simulink model "Controls"  (R2020b)
settings: Solver=VariableStepAuto  StartTime=0.0  StopTime=30  RelTol=1e-3
model workspace (MAT data in the model file):
  l1 = Simulink.Parameter
  l1.Value = 0.2
  l1.Description = '"Bicep length"'
  l1.DataType = 'auto'
  l1.Dimensions = [1 1]
  l2 = Simulink.Parameter
  l2.Value = 0.15
  l2.Description = '"Forearm length"'
  l2.DataType = 'auto'
  l2.Dimensions = [1 1]
settings Model: PacingRate=0.500000  OrderedModelArguments=off  Creator=Luke Bidulka  LastModifiedBy=ndroz

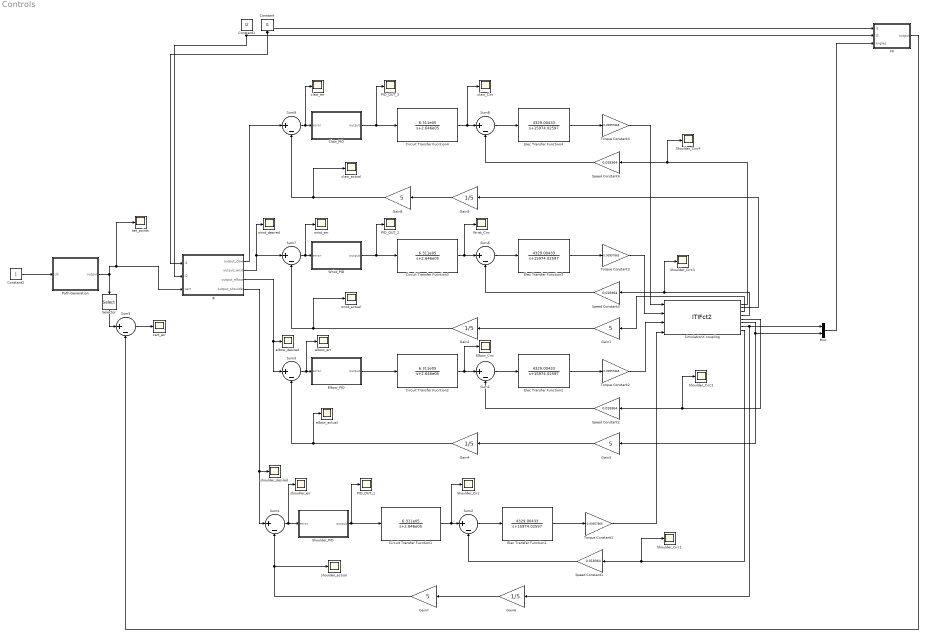
== system Controls ==
  Circuit Transfer Fucntion{1..4} (4 alike) : TransferFcn  Numerator=[6.311e05]  Denominator=[1 2.646e05]
  Claw_PID : MATLAB Function  TreatAsAtomicUnit=on  SystemSampleTime=0.001
  Constant : Constant  Value=l1
  Constant1 : Constant  Value=l2
  Constant2 : Constant  SampleTime=0.001
  Elbow_Circ : Scope
  Elbow_PID : MATLAB Function  TreatAsAtomicUnit=on  SystemSampleTime=0.001
  Elec Transfer Function{1..4} (4 alike) : TransferFcn  Numerator=[4329.00433]  Denominator=[1 15974.02597]
  FK : MATLAB Function  TreatAsAtomicUnit=on
  Gain{1,3,7..8} (4 alike) : Gain  Gain=5
  Gain{2,4..6} (4 alike) : Gain  Gain=1/5
  IK : MATLAB Function  TreatAsAtomicUnit=on  SystemSampleTime=0.001
  Mux : Mux  Inputs=2
  PID_OUT_1 : Scope
  PID_OUT_2 : Scope
  PID_OUT_3 : Scope
  Path Generation : MATLAB Function  TreatAsAtomicUnit=on
  Selector : Selector  InputPortWidth=3  IndexOptions=Index vector (dialog)  Indices=[1 2]  OutputSizes=1
  Shoulder_Circ{,1..4} (5 alike) : Scope
  Shoulder_PID : MATLAB Function  TreatAsAtomicUnit=on  SystemSampleTime=0.001
  SimulationX coupling : S-Function  FunctionName=ITIFct2  Parameters=ip, port, ts, nIn, nOut  SFunctionDeploymentMode=off  EnableBusSupport=off  mask{ip='localhost', port=4098, ts=0.001, nIn=4, nOut=8}
      mask prompts: ip "Address: ip"; port "Port Number: port [-]"; ts "Communication Step Size: ts [s]"; nIn "Input Vector Dimension (to SimulationX): nIn [-]"; nOut "Output Vector Dimension (from SimulationX): nOut [-]"
      mask help: Coupling Element
  Speed Constant{1..4} (4 alike) : Gain  Gain=0.018364
  Sum{1..9} (9 alike) : Sum  Inputs=|+-
  Torque Constant{1..4} (4 alike) : Gain  Gain=0.00957865
  Wrist_Circ : Scope
  Wrist_PID : MATLAB Function  TreatAsAtomicUnit=on  SystemSampleTime=0.001
  cart_err : Scope
  claw_Circ : Scope
  claw_actual : Scope
  claw_err : Scope
  elbow_actual : Scope
  elbow_desired : Scope
  elbow_err : Scope
  set_points : Scope
  shoudler_err : Scope
  shoulder_actual : Scope
  shoulder_desired : Scope
  wrist_actual : Scope
  wrist_desired : Scope
  wrist_err : Scope
  wires:
  Path Generation/1(output) -> set_points/1, IK/3(cart), Selector/1
  Constant1/1 -> IK/2(l2), FK/2(l2)
  Constant/1 -> IK/1(l1), FK/1(l1)
  Elec Transfer Function1/1 -> Torque Constant1/1
  Circuit Transfer Fucntion1/1 -> Shoulder_Circ/1, Sum2/1
  Sum2/1 -> Elec Transfer Function1/1
  Elec Transfer Function2/1 -> Torque Constant2/1
  Speed Constant2/1 -> Sum1/2
  Gain3/1 -> Gain4/1
  Sum1/1 -> Elec Transfer Function2/1
  Circuit Transfer Fucntion2/1 -> Elbow_Circ/1, Sum1/1
  Gain4/1 -> Sum3/2, elbow_actual/1
  IK/3(output_elbow) -> Sum3/1, elbow_desired/1
  Mux/1 -> FK/3(angles)
  Gain6/1 -> Gain7/1
  Sum5/1 -> cart_err/1
  Shoulder_PID/1(output) -> Circuit Transfer Fucntion1/1, PID_OUT_1/1
  Constant2/1 -> Path Generation/1(clk)
  Elbow_PID/1(output) -> Circuit Transfer Fucntion2/1
  Sum3/1 -> elbow_err/1, Elbow_PID/1(error)
  IK/4(output_shoulder) -> Sum4/1, shoulder_desired/1
  Sum4/1 -> shoudler_err/1, Shoulder_PID/1(error)
  Sum7/1 -> wrist_err/1, Wrist_PID/1(error)
  Wrist_PID/1(output) -> Circuit Transfer Fucntion3/1, PID_OUT_2/1
  Sum6/1 -> Elec Transfer Function3/1
  Circuit Transfer Fucntion3/1 -> Wrist_Circ/1, Sum6/1
  Gain2/1 -> Sum7/2, wrist_actual/1
  Elec Transfer Function3/1 -> Torque Constant3/1
  Gain1/1 -> Gain2/1
  Speed Constant3/1 -> Sum6/2
  IK/2(output_wrist) -> wrist_desired/1, Sum7/1
  Gain7/1 -> Sum4/2, shoulder_actual/1
  Speed Constant1/1 -> Sum2/2
  Gain8/1 -> Sum9/2, claw_actual/1
  Speed Constant4/1 -> Sum8/2
  Claw_PID/1(output) -> Circuit Transfer Fucntion4/1, PID_OUT_3/1
  Circuit Transfer Fucntion4/1 -> claw_Circ/1, Sum8/1
  Sum9/1 -> claw_err/1, Claw_PID/1(error)
  Sum8/1 -> Elec Transfer Function4/1
  Elec Transfer Function4/1 -> Torque Constant4/1
  Gain5/1 -> Gain8/1
  Torque Constant1/1 -> SimulationX coupling/4
  Torque Constant2/1 -> SimulationX coupling/3
  Torque Constant3/1 -> SimulationX coupling/2
  SimulationX coupling/7 -> Mux/1, Gain6/1
  SimulationX coupling/6 -> Mux/2, Gain3/1
  SimulationX coupling/5 -> Shoulder_Circ2/1, Speed Constant2/1
  Torque Constant4/1 -> SimulationX coupling/1
  SimulationX coupling/4 -> Shoulder_Circ3/1, Speed Constant3/1
  SimulationX coupling/3 -> Gain1/1
  SimulationX coupling/1 -> Shoulder_Circ4/1, Speed Constant4/1
  SimulationX coupling/2 -> Gain5/1
  IK/1(output_claw) -> Sum9/1
  SimulationX coupling/8 -> Shoulder_Circ1/1, Speed Constant1/1
  FK/1(output) -> Sum5/2
  Selector/1 -> Sum5/1

== matlab function Controls/FK ==
  data: l1 input; l2 input; angles input; output output
% Fwd Kinematics
function output = Fwd_Kin(l1, l2, angles)

    q0 = angles(1) / 35; % Configuration-space shoulder angle
    q1 = angles(2) / 35; % Configuration-space elbow angle

    % Get task-space coordinates
    x = l1*cos(q0) + l2*cos(q0+q1);
    y = l1*sin(q0) + l2*sin(q0+q1);

    % Output the task-space cartesian coordinats
    output = [x;y];

end

== matlab function Controls/IK ==
  data: output_claw output; output_wrist output; output_elbow output; l1 input; l2 input; cart input; output_shoulder output
% Inv Kinematics
function [output_claw,output_wrist,output_elbow,output_shoulder] = Inv_Kin(l1, l2, cart)
    x = cart(1); % Task-space x coord
    y = cart(2); % Task-space y coord
    
    % Get q1 first, need it to calculate q0. We will always
    % take the "right-handed" solution where q1 is (+). 
    q1 = abs(acos((x^2 + y^2 - l1^2 - l2^2)/(2*l1*l2)));

    % Get q0
    gamma = atan(y/x);
    beta = atan((l2*sin(q1))/(l1 + l2*cos(q1)));

    q0 = gamma - beta;
    
    % Ouput our angle vector
    if cart(3) == 0
        output_claw = -0.6;
    else
        output_claw = 0.3;
    end
    output_wrist = 35 * (-q0 - q1 + 70*(2*3.1415/360));
    output_elbow = 35 * q1;
    output_shoulder = 35 * q0;
    
end

== matlab function Controls/Path Generation ==
  settings: sampleTime=0.2
  data: output output; clk input
function output  = path_gen(clk)
    persistent count path_points path_size
    
    if isempty(count)
        count = 1;
        path_points = generate_path();
        path_size = length(path_points);
    end
    
    if clk == 1
        if count ~= path_size
            count = count + 1;
        end
    end
    
    output = path_points(count,:);
end

function output = generate_path()
    persistent count event event_count array_position x_value x_value_increment

    t = (0:0.1:50)'; % Time
    wait_length = 500;
    claw_open = 0;
    claw_close = 1;
    claw_old_state = claw_open;
    idle = 0;
    first_marsh = 1;
    first_marsh_idle = 2;
    second_marsh = 3;
    second_marsh_idle = 4;
    third_marsh = 5;
    third_marsh_idle = 6;
    garbage = 7;
    table_length = 0.3;
    table_angle = 70;
    table_origin = [0.15 0.30];
    gripper_len = 0.098;
    gripper_adjustment = 0.01;
    
    current_point = [0 0]; %Initialize
    next_point = [0 0]; %Initialize
    starting_point = [0.2 0.15];
    first_marsh_point = [table_origin(1)-table_length/4*sind(table_angle)-gripper_adjustment*sind(table_angle)-gripper_len*sind(90-table_angle) table_origin(2)+table_length/4*cosd(table_angle)+gripper_adjustment*cosd(table_angle)-gripper_len*cosd(90-table_angle)];
    second_marsh_point = [table_origin(1)-gripper_adjustment*sind(table_angle)-gripper_len*sind(90-table_angle) table_origin(2)+gripper_adjustment*cosd(table_angle)-gripper_len*cosd(90-table_angle)];
    third_marsh_point = [table_origin(1)+table_length/4*sind(table_angle)-gripper_adjustment*sind(table_angle)-gripper_len*sind(90-table_angle) table_origin(2)-table_length/4*cosd(table_angle)+gripper_adjustment*cosd(table_angle)-gripper_len*cosd(90-table_angle)];
    first_garbage_point = [first_marsh_point(1)-0.1*sind(90-table_angle) first_marsh_point(2)-0.1*cosd(90-table_angle)];
    second_garbage_point = [second_marsh_point(1)-0.1*sind(90-table_angle) second_marsh_point(2)-0.1*cosd(90-table_angle)];
    third_garbage_point = [third_marsh_point(1)-0.1*sind(90-table_angle) third_marsh_point(2)-0.1*cosd(90-table_angle)];

    path_vector = [garbage first_marsh_idle first_marsh garbage second_marsh_idle second_marsh garbage third_marsh_idle third_marsh garbage idle];
    path_points = zeros(100000,3);
    
    if isempty(count)
        event_count = 1;
        count = 1;
        array_position = 1;
        x_value_increment = 0.005;
    end
    
    while event_count <= length(path_vector)
        event = path_vector(event_count);
        x_value = 8;

        switch event
            case garbage 
                if event_count == 1
                    current_point = starting_point;
                    next_point = second_garbage_point;
                elseif path_vector(event_count - 1) == first_marsh
                    current_point = first_marsh_point;
                    next_point = first_garbage_point;
                elseif path_vector(event_count - 1) == second_marsh
                    current_point = second_marsh_point;
                    next_point = second_garbage_point;
                else 
                    current_point = third_marsh_point;
                    next_point = third_garbage_point;
                end
            case first_marsh_idle
                current_point = second_garbage_point;
                next_point = first_garbage_point;
            case first_marsh
                current_point = first_garbage_point;
                next_point = first_marsh_point;
            case second_marsh_idle
                current_point = first_garbage_point;
                next_point = second_garbage_point; 
            case second_marsh 
                current_point = second_garbage_point;
                next_point = second_marsh_point;
            case third_marsh_idle
                current_point = second_garbage_point;
                next_point = third_garbage_point; 
            case third_marsh
                current_point = third_garbage_point;
                next_point = third_marsh_point;
            case idle
                current_point = third_garbage_point;
                next_point = second_garbage_point;
        end

        x_point = current_point(1);
        y_point = current_point(2);
        

        while ((abs(x_point - current_point(1)) <= abs(next_point(1) - current_point(1))) && (abs(y_point - current_point(2)) <= abs(next_point(2) - current_point(2))))
            if (event == first_marsh || event == second_marsh || event == third_marsh)
                increment_x = (next_point(1) - current_point(1)) / (1*(x_value^3));
                increment_y = (next_point(2) - current_point(2)) / (1*(x_value^3));
                if (1*(x_value^3) < 5000)
                    x_value = x_value + x_value_increment;
                end
            else
                increment_x = (next_point(1) - current_point(1)) / length(t);
                increment_y = (next_point(2) - current_point(2)) / length(t);
            end
            x_point = x_point + increment_x;
            y_point = y_point + increment_y;
            path_points(array_position,:) = [x_point y_point claw_old_state];
            array_position = array_position + 1;
        end   

        for i = 1:wait_length
            if (event == first_marsh || event == second_marsh || event == third_marsh) && (i > wait_length/2)
                path_points(array_position,:) = [x_point y_point claw_close];
                claw_old_state = claw_close;
            elseif (event == garbage) && (i > wait_length/2)
                path_points(array_position,:) = [x_point y_point claw_open];
                claw_old_state = claw_open;
            else
                path_points(array_position,:) = [x_point y_point claw_old_state];
            end
            array_position = array_position + 1;
        end

        event_count = event_count +1;
    end
    
    path_points(array_position:end, :) = [];
    output = path_points;
end

== matlab function Controls/Shoulder_PID ==
  data: error input; output output
function output = PID(error)
    persistent pid_integrator pid_prev_error pid_lim_min pid_lim_max sample_time Kp Ki Kd Tau diff_array diff_mult
    if isempty(pid_integrator)
        pid_integrator = 0;
        pid_prev_error = 0;
        pid_lim_min = -5;
        pid_lim_max = 5;
        sample_time = 0.001;
        Kp = 3; %15;
        Ki = 0.001; %1;
        Kd = 0.2574; %0.85;
        Tau = 600;
        diff_array = zeros(1,4);
        diff_mult = [exp(-Tau)^(7*sample_time/2) exp(-Tau)^(5*sample_time/2) exp(-Tau)^(3*sample_time/2) exp(-Tau)^(sample_time/2)];
    end

    %Proportional
    proportional = Kp*error;

    %Integral
    pid_integrator = pid_integrator + 0.5*Ki*sample_time*(error + pid_prev_error);

    %Derivative
    diff_array(4) = Kd*(error - pid_prev_error)/sample_time;
    pid_differentiator = 0;
    for i = 1:length(diff_array)
       pid_differentiator = pid_differentiator + (diff_array(i)*diff_mult(i));
    end

    diff_array = circshift(diff_array,[0, -1]);
    pid_prev_error = error; 
    
    output = proportional + pid_integrator + pid_differentiator;
    
    if output > pid_lim_max
       output = pid_lim_max;
    elseif output < pid_lim_min
       output = pid_lim_min;
    end
end

== matlab function Controls/Elbow_PID ==
  data: error input; output output
function output = PID(error)
    persistent pid_integrator pid_prev_error pid_lim_min pid_lim_max sample_time Kp Ki Kd Tau diff_array diff_mult
    if isempty(pid_integrator)
        pid_integrator = 0;
        pid_prev_error = 0;
        pid_lim_min = -5;
        pid_lim_max = 5;
        sample_time = 0.001;
        Kp = 2.2; %2.2
        Ki = 0;
        Kd = 0.11; %0.1
        Tau = 600;
        diff_array = zeros(1,4);
        diff_mult = [exp(-Tau)^(7*sample_time/2) exp(-Tau)^(5*sample_time/2) exp(-Tau)^(3*sample_time/2) exp(-Tau)^(sample_time/2)];
    end

    %Proportional
    proportional = Kp*error;

    %Integral
    pid_integrator = pid_integrator + 0.5*Ki*sample_time*(error + pid_prev_error);

    %Derivative
    diff_array(4) = Kd*(error - pid_prev_error)/sample_time;
    pid_differentiator = 0;
    for i = 1:length(diff_array)
       pid_differentiator = pid_differentiator + (diff_array(i)*diff_mult(i));
    end

    diff_array = circshift(diff_array,[0, -1]);
    pid_prev_error = error; 
    
    output = proportional + pid_integrator + pid_differentiator;
    
    if output > pid_lim_max
       output = pid_lim_max;
    elseif output < pid_lim_min
       output = pid_lim_min;
    end
end

== matlab function Controls/Wrist_PID ==
  data: error input; output output
function output = PID(error)
    persistent pid_integrator pid_prev_error pid_lim_min pid_lim_max sample_time Kp Ki Kd Tau diff_array diff_mult
    if isempty(pid_integrator)
        pid_integrator = 0;
        pid_prev_error = 0;
        pid_lim_min = -5.2;
        pid_lim_max = 5.2;
        sample_time = 0.001;
        Kp = 1; %1
        Ki = 0.00007;
        Kd = 0.03; %0.03
        Tau = 600;
        diff_array = zeros(1,4);
        diff_mult = [exp(-Tau)^(7*sample_time/2) exp(-Tau)^(5*sample_time/2) exp(-Tau)^(3*sample_time/2) exp(-Tau)^(sample_time/2)];
    end

    %Proportional
    proportional = Kp*error;

    %Integral
    pid_integrator = pid_integrator + 0.5*Ki*sample_time*(error + pid_prev_error);

    %Derivative
    diff_array(4) = Kd*(error - pid_prev_error)/sample_time;
    pid_differentiator = 0;
    for i = 1:length(diff_array)
       pid_differentiator = pid_differentiator + (diff_array(i)*diff_mult(i));
    end

    diff_array = circshift(diff_array,[0, -1]);
    pid_prev_error = error; 
    
    output = proportional + pid_integrator + pid_differentiator;
    
    if output > pid_lim_max
       output = pid_lim_max;
    elseif output < pid_lim_min
       output = pid_lim_min;
    end
end

== matlab function Controls/Claw_PID ==
  data: error input; output output
function output = PID(error)
    persistent pid_integrator pid_prev_error pid_lim_min pid_lim_max sample_time Kp Ki Kd Tau diff_array diff_mult
    if isempty(pid_integrator)
        pid_integrator = 0;
        pid_prev_error = 0;
        pid_lim_min = -5;
        pid_lim_max = 5;
        sample_time = 0.001;
        Kp = 81; %15;
        Ki = 0; %0.1;
        Kd = 2; %0.85;
        Tau = 600;
        diff_array = zeros(1,4);
        diff_mult = [exp(-Tau)^(7*sample_time/2) exp(-Tau)^(5*sample_time/2) exp(-Tau)^(3*sample_time/2) exp(-Tau)^(sample_time/2)];
    end

    %Proportional
    proportional = Kp*error;

    %Integral
    pid_integrator = pid_integrator + 0.5*Ki*sample_time*(error + pid_prev_error);

    %Derivative
    diff_array(4) = Kd*(error - pid_prev_error)/sample_time;
    pid_differentiator = 0;
    for i = 1:length(diff_array)
       pid_differentiator = pid_differentiator + (diff_array(i)*diff_mult(i));
    end

    diff_array = circshift(diff_array,[0, -1]);
    pid_prev_error = error; 
    
    output = proportional + pid_integrator + pid_differentiator;
    
    if output > pid_lim_max
       output = pid_lim_max;
    elseif output < pid_lim_min
       output = pid_lim_min;
    end
end
